simulink library "stimer_slib"  (R2014b)
settings: Solver=ode45  SolverMode=SingleTasking  StartTime=0.0  StopTime=10.0  RelTol=1e-3
undefined symbols (not defined in the file or in its folder): fx_stimer_ctrl, struct2array
settings Model: CovMetricSettings=dwe  CovHtmlReporting=off  CovSaveCumulativeToWorkspaceVar=off  CovSaveSingleToWorkspaceVar=off  CovExternalEMLEnable=on  CovSFcnEnable=on  Creator=LCD  LastModifiedBy=Camilo

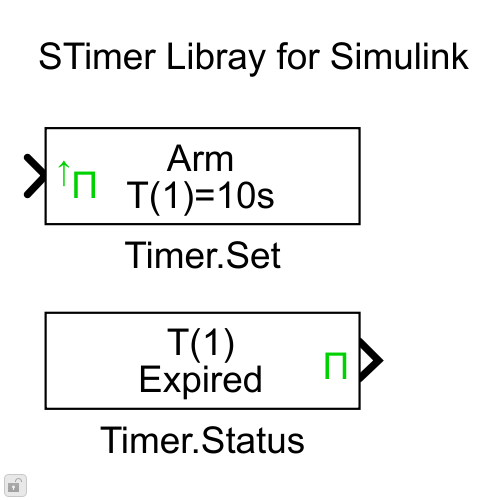
[thumbnail: Simulink's stored preview of the top-level diagram]
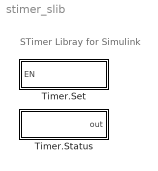
== system stimer_slib ==
  note: STimer Libray for Simulink
  Timer.Set : Subsystem  mask(Timer.Set){tindex=1, tvalue=10}
      mask prompts: tindex "Timer index ( 1 to 256 )"; tvalue "Time value (seconds)"
      mask help:
      | Arms the selected timer by setting the provided time value.
      | A zero(0) time value will disarm the timer.
      | Action executes each time the control signal control signal rises from a negative or zero value to a positive value (rising edge). If the initial value is negative, a rising signal to zero triggers execution.
      mask Display:
      | if str2num(get_param(gcb,'tvalue'))>0
      |     fprintf('Arm\nT(%s)=%ss',get_param(gcb,'tindex'),get_param(gcb,'tvalue'))
      | else
      |     fprintf('Disarm\nT(%s)',get_param(gcb,'tindex'));
      | end
      | color('green')
      | port_label('input',1,'^{\uparrow}\Pi','texmode','on');
  Timer.Status : Subsystem  mask(Timer status){xtimer=1, prop=Expired}
      mask prompts: xtimer "Timer index ( 1 to 256 )"; prop "Requested status"
      mask help: Retrieve the status of the selected timer
      mask init:
      | % set_param(gcb, 'backgroundcolor','white')
      mask TypeOptions prop: Expired | Elapsed | Remaining
      mask Display:
      | fprintf('T(%s)\n%s',get_param(gcb,'xtimer'),get_param(gcb,'prop'));
      | switch get_param(gcb,'prop')
      |     case 'Expired'
      |         color('green');
      |         port_label('output',1,'\Pi','texmode','on');
      |     case 'Elapsed'
      |         color('blue');
      |         port_label('output',1,'\tau^E','texmode','on');
      |     case 'Remaining'
      |         color('blue');
      |         port_label('output',1,'\tau^R','texmode','on');
      | end

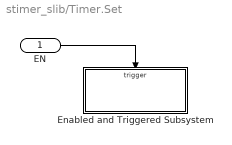
== system stimer_slib/Timer.Set ==
  EN : Inport
  Enabled and Triggered Subsystem : Subsystem  TreatAsAtomicUnit=on
  wires:
  EN/1 -> Enabled and Triggered Subsystem/Trigger

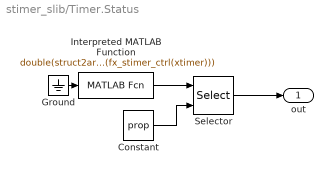
== system stimer_slib/Timer.Status ==
  Constant : Constant  Value=prop
  Ground : Ground
  Interpreted MATLAB Function : MATLABFcn  MATLABFcn=double(struct2array(fx_stimer_ctrl(xtimer)))  OutputDimensions=4  OutputSignalType=real
  Selector : Selector  InputPortWidth=4  IndexOptions=Starting index (port)  Indices=[1 3]  OutputSizes=1
  out : Outport
  wires:
  Ground/1 -> Interpreted MATLAB Function/1
  Selector/1 -> out/1
  Interpreted MATLAB Function/1 -> Selector/1
  Constant/1 -> Selector/2

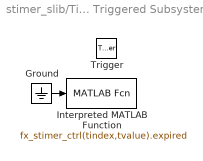
== system stimer_slib/Timer.Set/Enabled and Triggered Subsystem ==
  Trigger : TriggerPort
  Ground : Ground
  Interpreted MATLAB Function : MATLABFcn  MATLABFcn=fx_stimer_ctrl(tindex,tvalue).expired  OutputDimensions=0
  wires:
  Ground/1 -> Interpreted MATLAB Function/1
